simulink model "ques5"  (R2022b)
settings: Solver=ode4  StartTime=0.0  StopTime=10.0  FixedStep=0.0001  MaxStep=0.0001  RelTol=1e-3
values from neighbouring files (symbols this model uses):
  A = [a-b, 0.5-c; 0, 1]    [A2_2_4.m]    (also in A2_2_4_fin.m; A2_3_4_fin.m; A2_4_2.m = [a-bl, 0.5-c; 0, 1]; KA2_4.m = [a-bl, 0.5-c; 0, 1])
  B = [0; 1]    [A2_2_4.m]    (also in A2_2_4_fin.m; A2_3_4_fin.m; A2_4_2.m; KA2_4.m)
undefined symbols (not defined in the file or in its folder): C, D
settings Model: Creator=long  LastModifiedBy=munjunhwi
settings SolverCC: AlgebraicLoopSolver=TrustRegion
settings DebuggingCC: UnconnectedInputMsg=warning  UnconnectedOutputMsg=warning  UnconnectedLineMsg=warning  SFMachineParentedDataDiag=warning
settings ModelReferenceCC: EnableRefExpFcnMdlSchedulingChecks=on
settings RTWCC: DLArmComputeVersion=19.05

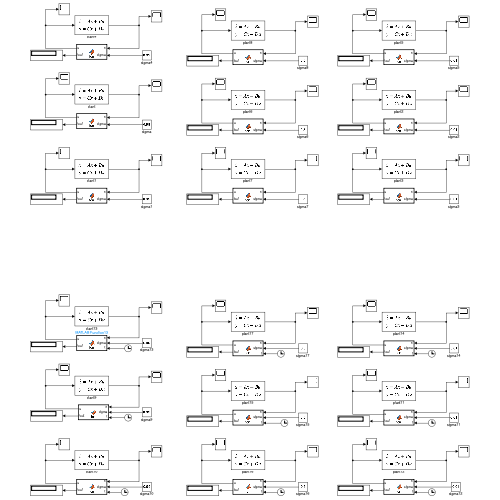
[thumbnail: Simulink's stored preview of the top-level diagram]
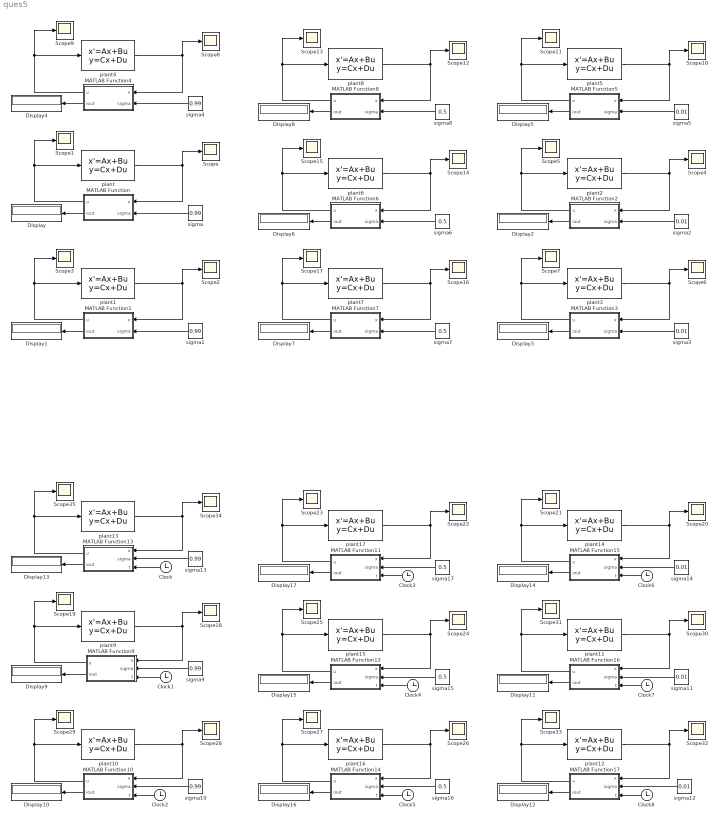
== system ques5 ==
  Clock{,1..8} (9 alike) : Clock
  Display{,1..17} (18 alike) : Display
  MATLAB Function : MATLAB Function  TreatAsAtomicUnit=on
  MATLAB Function1 : MATLAB Function  TreatAsAtomicUnit=on
  MATLAB Function10 : MATLAB Function  TreatAsAtomicUnit=on
  MATLAB Function11 : MATLAB Function  TreatAsAtomicUnit=on
  MATLAB Function12 : MATLAB Function  TreatAsAtomicUnit=on
  MATLAB Function13 : MATLAB Function  TreatAsAtomicUnit=on
  MATLAB Function14 : MATLAB Function  TreatAsAtomicUnit=on
  MATLAB Function15 : MATLAB Function  TreatAsAtomicUnit=on
  MATLAB Function16 : MATLAB Function  TreatAsAtomicUnit=on
  MATLAB Function17 : MATLAB Function  TreatAsAtomicUnit=on
  MATLAB Function2 : MATLAB Function  TreatAsAtomicUnit=on
  MATLAB Function3 : MATLAB Function  TreatAsAtomicUnit=on
  MATLAB Function4 : MATLAB Function  TreatAsAtomicUnit=on
  MATLAB Function5 : MATLAB Function  TreatAsAtomicUnit=on
  MATLAB Function6 : MATLAB Function  TreatAsAtomicUnit=on
  MATLAB Function7 : MATLAB Function  TreatAsAtomicUnit=on
  MATLAB Function8 : MATLAB Function  TreatAsAtomicUnit=on
  MATLAB Function9 : MATLAB Function  TreatAsAtomicUnit=on
  Scope{,1..35} (36 alike) : Scope
  plant{,2,6,9,11,15} (6 alike) : StateSpace  A=A  B=B  C=C  D=D  InitialCondition=[10;10]
  plant{1,3,7,10,12,16} (6 alike) : StateSpace  A=A  B=B  C=C  D=D  InitialCondition=[1;0]
  plant{4..5,8,13..14,17} (6 alike) : StateSpace  A=A  B=B  C=C  D=D  InitialCondition=[100;150]
  sigma{,1,4,9..10,13} (6 alike) : Constant  Value=0.99
  sigma{2..3,5,11..12,14} (6 alike) : Constant  Value=0.01
  sigma{6..8,15..17} (6 alike) : Constant  Value=0.5
  wires:
  sigma/1 -> MATLAB Function/2(sigma)
  plant/1 -> MATLAB Function/1(x), Scope/1
  MATLAB Function/1(u) -> Scope1/1, plant/1
  MATLAB Function/2(iout) -> Display/1
  MATLAB Function1/2(iout) -> Display1/1
  MATLAB Function1/1(u) -> Scope3/1, plant1/1
  sigma1/1 -> MATLAB Function1/2(sigma)
  plant1/1 -> MATLAB Function1/1(x), Scope2/1
  MATLAB Function2/2(iout) -> Display2/1
  MATLAB Function2/1(u) -> Scope5/1, plant2/1
  sigma2/1 -> MATLAB Function2/2(sigma)
  plant2/1 -> MATLAB Function2/1(x), Scope4/1
  MATLAB Function3/2(iout) -> Display3/1
  MATLAB Function3/1(u) -> Scope7/1, plant3/1
  sigma3/1 -> MATLAB Function3/2(sigma)
  plant3/1 -> MATLAB Function3/1(x), Scope6/1
  sigma5/1 -> MATLAB Function5/2(sigma)
  MATLAB Function5/1(u) -> Scope11/1, plant5/1
  MATLAB Function4/2(iout) -> Display4/1
  MATLAB Function4/1(u) -> Scope9/1, plant4/1
  sigma4/1 -> MATLAB Function4/2(sigma)
  plant5/1 -> MATLAB Function5/1(x), Scope10/1
  MATLAB Function5/2(iout) -> Display5/1
  plant4/1 -> MATLAB Function4/1(x), Scope8/1
  sigma6/1 -> MATLAB Function6/2(sigma)
  MATLAB Function6/1(u) -> Scope15/1, plant6/1
  plant6/1 -> MATLAB Function6/1(x), Scope14/1
  MATLAB Function8/1(u) -> Scope13/1, plant8/1
  MATLAB Function8/2(iout) -> Display8/1
  plant8/1 -> MATLAB Function8/1(x), Scope12/1
  MATLAB Function6/2(iout) -> Display6/1
  sigma8/1 -> MATLAB Function8/2(sigma)
  sigma7/1 -> MATLAB Function7/2(sigma)
  MATLAB Function7/1(u) -> Scope17/1, plant7/1
  plant7/1 -> MATLAB Function7/1(x), Scope16/1
  MATLAB Function7/2(iout) -> Display7/1
  sigma11/1 -> MATLAB Function16/2(sigma)
  MATLAB Function16/1(u) -> Scope31/1, plant11/1
  plant11/1 -> MATLAB Function16/1(x), Scope30/1
  MATLAB Function10/2(iout) -> Display10/1
  sigma10/1 -> MATLAB Function10/2(sigma)
  plant10/1 -> MATLAB Function10/1(x), Scope28/1
  MATLAB Function15/1(u) -> Scope21/1, plant14/1
  MATLAB Function13/2(iout) -> Display13/1
  MATLAB Function13/1(u) -> Scope35/1, plant13/1
  plant14/1 -> MATLAB Function15/1(x), Scope20/1
  MATLAB Function16/2(iout) -> Display11/1
  MATLAB Function17/1(u) -> Scope33/1, plant12/1
  sigma12/1 -> MATLAB Function17/2(sigma)
  MATLAB Function17/2(iout) -> Display12/1
  plant12/1 -> MATLAB Function17/1(x), Scope32/1
  MATLAB Function14/2(iout) -> Display16/1
  plant16/1 -> MATLAB Function14/1(x), Scope26/1
  MATLAB Function12/2(iout) -> Display15/1
  sigma16/1 -> MATLAB Function14/2(sigma)
  plant17/1 -> MATLAB Function11/1(x), Scope22/1
  sigma14/1 -> MATLAB Function15/2(sigma)
  MATLAB Function14/1(u) -> Scope27/1, plant16/1
  MATLAB Function10/1(u) -> Scope29/1, plant10/1
  plant15/1 -> MATLAB Function12/1(x), Scope24/1
  MATLAB Function12/1(u) -> Scope25/1, plant15/1
  sigma13/1 -> MATLAB Function13/2(sigma)
  MATLAB Function11/2(iout) -> Display17/1
  MATLAB Function11/1(u) -> Scope23/1, plant17/1
  sigma17/1 -> MATLAB Function11/2(sigma)
  MATLAB Function9/1(u) -> Scope19/1, plant9/1
  MATLAB Function9/2(iout) -> Display9/1
  MATLAB Function15/2(iout) -> Display14/1
  sigma9/1 -> MATLAB Function9/2(sigma)
  plant9/1 -> MATLAB Function9/1(x), Scope18/1
  sigma15/1 -> MATLAB Function12/2(sigma)
  plant13/1 -> MATLAB Function13/1(x), Scope34/1
  Clock/1 -> MATLAB Function13/3(t)
  Clock1/1 -> MATLAB Function9/3(t)
  Clock2/1 -> MATLAB Function10/3(t)
  Clock3/1 -> MATLAB Function11/3(t)
  Clock4/1 -> MATLAB Function12/3(t)
  Clock5/1 -> MATLAB Function14/3(t)
  Clock6/1 -> MATLAB Function15/3(t)
  Clock7/1 -> MATLAB Function16/3(t)
  Clock8/1 -> MATLAB Function17/3(t)

== matlab function ques5/MATLAB Function10 ==
  settings: updateMethod=DISCRETE
  data: x input; u output; sigma input; iout output; t input
function [u,iout]= fcn(x,sigma,t)
    persistent uk xk i;
    k1=zeros(1,2);
    A=zeros(2);
    B=zeros(2,1);
    P=zeros(2);
    Q=zeros(2);
    coder.extrinsic('evalin');
    A = evalin('base', 'A'); 
    B = evalin('base', 'B'); 
    P = evalin('base', 'P'); 
    Q = evalin('base', 'Q'); 
    k1 = evalin('base', 'k1'); 
    
    
    if isempty(uk)||isempty(xk)
        i=0;
        xk = x;
        uk=-k1*x;
    end

    
    if rem(t,0.0035)==0
        if [x' xk']*[A'*P+P*A+sigma*Q -P*B*k1;-(B*k1)'*P zeros(2)]*[x;xk]>=0
            i = i+1;
            uk = -k1*x;
            xk = x;
        end
    end

    u=uk;
    iout=i;
end

== matlab function ques5/MATLAB Function11 ==
  settings: updateMethod=DISCRETE
  data: x input; u output; sigma input; iout output; t input
function [u,iout]= fcn(x,sigma,t)
    persistent uk xk i;
    k1=zeros(1,2);
    A=zeros(2);
    B=zeros(2,1);
    P=zeros(2);
    Q=zeros(2);
    coder.extrinsic('evalin');
    A = evalin('base', 'A'); 
    B = evalin('base', 'B'); 
    P = evalin('base', 'P'); 
    Q = evalin('base', 'Q'); 
    k1 = evalin('base', 'k1'); 
    
    
    if isempty(uk)||isempty(xk)
        i=0;
        xk = x;
        uk=-k1*x;
    end

    
    if rem(t,0.0035)==0
        if [x' xk']*[A'*P+P*A+sigma*Q -P*B*k1;-(B*k1)'*P zeros(2)]*[x;xk]>=0
            i = i+1;
            uk = -k1*x;
            xk = x;
        end
    end

    u=uk;
    iout=i;
end

== matlab function ques5/MATLAB Function13 ==
  settings: updateMethod=DISCRETE
  data: x input; u output; sigma input; iout output; t input
function [u,iout]= fcn(x,sigma,t)
    persistent uk xk i;
    k1=zeros(1,2);
    A=zeros(2);
    B=zeros(2,1);
    P=zeros(2);
    Q=zeros(2);
    coder.extrinsic('evalin');
    A = evalin('base', 'A'); 
    B = evalin('base', 'B'); 
    P = evalin('base', 'P'); 
    Q = evalin('base', 'Q'); 
    k1 = evalin('base', 'k1'); 
    
    
    if isempty(uk)||isempty(xk)
        i=0;
        xk = x;
        uk=-k1*x;
    end

    
    if rem(t,0.0035)==0 %sampling time 0.0035
        if [x' xk']*[A'*P+P*A+sigma*Q -P*B*k1;-(B*k1)'*P zeros(2)]*[x;xk]>=0
            i = i+1;
            uk = -k1*x;
            xk = x;
        end
    end

    u=uk;
    iout=i;
end

== matlab function ques5/MATLAB Function12 ==
  settings: updateMethod=DISCRETE
  data: x input; u output; sigma input; iout output; t input
function [u,iout]= fcn(x,sigma,t)
    persistent uk xk i;
    k1=zeros(1,2);
    A=zeros(2);
    B=zeros(2,1);
    P=zeros(2);
    Q=zeros(2);
    coder.extrinsic('evalin');
    A = evalin('base', 'A'); 
    B = evalin('base', 'B'); 
    P = evalin('base', 'P'); 
    Q = evalin('base', 'Q'); 
    k1 = evalin('base', 'k1'); 
    
    
    if isempty(uk)||isempty(xk)
        i=0;
        xk = x;
        uk=-k1*x;
    end

    
    if rem(t,0.0035)==0
        if [x' xk']*[A'*P+P*A+sigma*Q -P*B*k1;-(B*k1)'*P zeros(2)]*[x;xk]>=0
            i = i+1;
            uk = -k1*x;
            xk = x;
        end
    end

    u=uk;
    iout=i;
end

== matlab function ques5/MATLAB Function14 ==
  settings: updateMethod=DISCRETE
  data: x input; u output; sigma input; iout output; t input
function [u,iout]= fcn(x,sigma,t)
    persistent uk xk i;
    k1=zeros(1,2);
    A=zeros(2);
    B=zeros(2,1);
    P=zeros(2);
    Q=zeros(2);
    coder.extrinsic('evalin');
    A = evalin('base', 'A'); 
    B = evalin('base', 'B'); 
    P = evalin('base', 'P'); 
    Q = evalin('base', 'Q'); 
    k1 = evalin('base', 'k1'); 
    
    
    if isempty(uk)||isempty(xk)
        i=0;
        xk = x;
        uk=-k1*x;
    end

    
    if rem(t,0.0035)==0
        if [x' xk']*[A'*P+P*A+sigma*Q -P*B*k1;-(B*k1)'*P zeros(2)]*[x;xk]>=0
            i = i+1;
            uk = -k1*x;
            xk = x;
        end
    end

    u=uk;
    iout=i;
end

== matlab function ques5/MATLAB Function15 ==
  settings: updateMethod=DISCRETE
  data: x input; u output; sigma input; iout output; t input
function [u,iout]= fcn(x,sigma,t)
    persistent uk xk i;
    k1=zeros(1,2);
    A=zeros(2);
    B=zeros(2,1);
    P=zeros(2);
    Q=zeros(2);
    coder.extrinsic('evalin');
    A = evalin('base', 'A'); 
    B = evalin('base', 'B'); 
    P = evalin('base', 'P'); 
    Q = evalin('base', 'Q'); 
    k1 = evalin('base', 'k1'); 
    
    
    if isempty(uk)||isempty(xk)
        i=0;
        xk = x;
        uk=-k1*x;
    end

    
    if rem(t,0.0035)==0
        if [x' xk']*[A'*P+P*A+sigma*Q -P*B*k1;-(B*k1)'*P zeros(2)]*[x;xk]>=0
            i = i+1;
            uk = -k1*x;
            xk = x;
        end
    end

    u=uk;
    iout=i;
end

== matlab function ques5/MATLAB Function1 ==
  settings: updateMethod=DISCRETE
  data: x input; u output; sigma input; iout output
function [u,iout]= fcn(x,sigma)
    persistent uk xk i;
    k1=zeros(1,2);
    A=zeros(2);
    B=zeros(2,1);
    P=zeros(2);
    Q=zeros(2);
    coder.extrinsic('evalin');
    A = evalin('base', 'A'); 
    B = evalin('base', 'B'); 
    P = evalin('base', 'P'); 
    Q = evalin('base', 'Q'); 
    k1 = evalin('base', 'k1'); 
    
    
    if isempty(uk)||isempty(xk)
        i=0;
        xk = x;
        uk=-k1*x;
    end

    if [x' xk']*[A'*P+P*A+sigma*Q -P*B*k1;-(B*k1)'*P zeros(2)]*[x;xk]>=0
        i = i+1;
        uk = -k1*x;
        xk = x;
    end

    u=uk;
    iout=i;
end

== matlab function ques5/MATLAB Function16 ==
  settings: updateMethod=DISCRETE
  data: x input; u output; sigma input; iout output; t input
function [u,iout]= fcn(x,sigma,t)
    persistent uk xk i;
    k1=zeros(1,2);
    A=zeros(2);
    B=zeros(2,1);
    P=zeros(2);
    Q=zeros(2);
    coder.extrinsic('evalin');
    A = evalin('base', 'A'); 
    B = evalin('base', 'B'); 
    P = evalin('base', 'P'); 
    Q = evalin('base', 'Q'); 
    k1 = evalin('base', 'k1'); 
    
    
    if isempty(uk)||isempty(xk)
        i=0;
        xk = x;
        uk=-k1*x;
    end

    
    if rem(t,0.0035)==0
        if [x' xk']*[A'*P+P*A+sigma*Q -P*B*k1;-(B*k1)'*P zeros(2)]*[x;xk]>=0
            i = i+1;
            uk = -k1*x;
            xk = x;
        end
    end

    u=uk;
    iout=i;
end

== matlab function ques5/MATLAB Function17 ==
  settings: updateMethod=DISCRETE
  data: x input; u output; sigma input; iout output; t input
function [u,iout]= fcn(x,sigma,t)
    persistent uk xk i;
    k1=zeros(1,2);
    A=zeros(2);
    B=zeros(2,1);
    P=zeros(2);
    Q=zeros(2);
    coder.extrinsic('evalin');
    A = evalin('base', 'A'); 
    B = evalin('base', 'B'); 
    P = evalin('base', 'P'); 
    Q = evalin('base', 'Q'); 
    k1 = evalin('base', 'k1'); 
    
    
    if isempty(uk)||isempty(xk)
        i=0;
        xk = x;
        uk=-k1*x;
    end

    
    if rem(t,0.0035)==0
        if [x' xk']*[A'*P+P*A+sigma*Q -P*B*k1;-(B*k1)'*P zeros(2)]*[x;xk]>=0
            i = i+1;
            uk = -k1*x;
            xk = x;
        end
    end

    u=uk;
    iout=i;
end

== matlab function ques5/MATLAB Function ==
  settings: updateMethod=DISCRETE
  data: x input; u output; sigma input; iout output
function [u,iout]= fcn(x,sigma)
    persistent uk xk i;
    k1=zeros(1,2);
    A=zeros(2);
    B=zeros(2,1);
    P=zeros(2);
    Q=zeros(2);
    coder.extrinsic('evalin');
    A = evalin('base', 'A'); 
    B = evalin('base', 'B'); 
    P = evalin('base', 'P'); 
    Q = evalin('base', 'Q'); 
    k1 = evalin('base', 'k1'); 
    
    
    if isempty(uk)||isempty(xk)
        i=0;
        xk = x;
        uk=-k1*x;
    end

    if [x' xk']*[A'*P+P*A+sigma*Q -P*B*k1;-(B*k1)'*P zeros(2)]*[x;xk]>=0
        i = i+1;
        uk = -k1*x;
        xk = x;
    end

    u=uk;
    iout=i;
end

== matlab function ques5/MATLAB Function2 ==
  settings: updateMethod=DISCRETE
  data: x input; u output; sigma input; iout output
function [u,iout]= fcn(x,sigma)
    persistent uk xk i;
    k1=zeros(1,2);
    A=zeros(2);
    B=zeros(2,1);
    P=zeros(2);
    Q=zeros(2);
    coder.extrinsic('evalin');
    A = evalin('base', 'A'); 
    B = evalin('base', 'B'); 
    P = evalin('base', 'P'); 
    Q = evalin('base', 'Q'); 
    k1 = evalin('base', 'k1'); 
    
    
    if isempty(uk)||isempty(xk)
        i=0;
        xk = x;
        uk=-k1*x;
    end

    if [x' xk']*[A'*P+P*A+sigma*Q -P*B*k1;-(B*k1)'*P zeros(2)]*[x;xk]>=0
        i = i+1;
        uk = -k1*x;
        xk = x;
    end

    u=uk;
    iout=i;
end

== matlab function ques5/MATLAB Function3 ==
  settings: updateMethod=DISCRETE
  data: x input; u output; sigma input; iout output
function [u,iout]= fcn(x,sigma)
    persistent uk xk i;
    k1=zeros(1,2);
    A=zeros(2);
    B=zeros(2,1);
    P=zeros(2);
    Q=zeros(2);
    coder.extrinsic('evalin');
    A = evalin('base', 'A'); 
    B = evalin('base', 'B'); 
    P = evalin('base', 'P'); 
    Q = evalin('base', 'Q'); 
    k1 = evalin('base', 'k1'); 
    
    
    if isempty(uk)||isempty(xk)
        i=0;
        xk = x;
        uk=-k1*x;
    end

    if [x' xk']*[A'*P+P*A+sigma*Q -P*B*k1;-(B*k1)'*P zeros(2)]*[x;xk]>=0
        i = i+1;
        uk = -k1*x;
        xk = x;
    end

    u=uk;
    iout=i;
end

== matlab function ques5/MATLAB Function4 ==
  settings: updateMethod=DISCRETE
  data: x input; u output; sigma input; iout output
function [u,iout]= fcn(x,sigma)
    persistent uk xk i;
    k1=zeros(1,2);
    A=zeros(2);
    B=zeros(2,1);
    P=zeros(2);
    Q=zeros(2);
    coder.extrinsic('evalin');
    A = evalin('base', 'A'); 
    B = evalin('base', 'B'); 
    P = evalin('base', 'P'); 
    Q = evalin('base', 'Q'); 
    k1 = evalin('base', 'k1'); 
    
    
    if isempty(uk)||isempty(xk)
        i=0;
        xk = x;
        uk=-k1*x;
    end

    if [x' xk']*[A'*P+P*A+sigma*Q -P*B*k1;-(B*k1)'*P zeros(2)]*[x;xk]>=0
        i = i+1;
        uk = -k1*x;
        xk = x;
    end

    u=uk;
    iout=i;
end

== matlab function ques5/MATLAB Function5 ==
  settings: updateMethod=DISCRETE
  data: x input; u output; sigma input; iout output
function [u,iout]= fcn(x,sigma)
    persistent uk xk i;
    k1=zeros(1,2);
    A=zeros(2);
    B=zeros(2,1);
    P=zeros(2);
    Q=zeros(2);
    coder.extrinsic('evalin');
    A = evalin('base', 'A'); 
    B = evalin('base', 'B'); 
    P = evalin('base', 'P'); 
    Q = evalin('base', 'Q'); 
    k1 = evalin('base', 'k1'); 
    
    
    if isempty(uk)||isempty(xk)
        i=0;
        xk = x;
        uk=-k1*x;
    end

    if [x' xk']*[A'*P+P*A+sigma*Q -P*B*k1;-(B*k1)'*P zeros(2)]*[x;xk]>=0
        i = i+1;
        uk = -k1*x;
        xk = x;
    end

    u=uk;
    iout=i;
end

== matlab function ques5/MATLAB Function6 ==
  settings: updateMethod=DISCRETE
  data: x input; u output; sigma input; iout output
function [u,iout]= fcn(x,sigma)
    persistent uk xk i;
    k1=zeros(1,2);
    A=zeros(2);
    B=zeros(2,1);
    P=zeros(2);
    Q=zeros(2);
    coder.extrinsic('evalin');
    A = evalin('base', 'A'); 
    B = evalin('base', 'B'); 
    P = evalin('base', 'P'); 
    Q = evalin('base', 'Q'); 
    k1 = evalin('base', 'k1'); 
    
    
    if isempty(uk)||isempty(xk)
        i=0;
        xk = x;
        uk=-k1*x;
    end

    if [x' xk']*[A'*P+P*A+sigma*Q -P*B*k1;-(B*k1)'*P zeros(2)]*[x;xk]>=0
        i = i+1;
        uk = -k1*x;
        xk = x;
    end

    u=uk;
    iout=i;
end

== matlab function ques5/MATLAB Function7 ==
  settings: updateMethod=DISCRETE
  data: x input; u output; sigma input; iout output
function [u,iout]= fcn(x,sigma)
    persistent uk xk i;
    k1=zeros(1,2);
    A=zeros(2);
    B=zeros(2,1);
    P=zeros(2);
    Q=zeros(2);
    coder.extrinsic('evalin');
    A = evalin('base', 'A'); 
    B = evalin('base', 'B'); 
    P = evalin('base', 'P'); 
    Q = evalin('base', 'Q'); 
    k1 = evalin('base', 'k1'); 
    
    
    if isempty(uk)||isempty(xk)
        i=0;
        xk = x;
        uk=-k1*x;
    end

    if [x' xk']*[A'*P+P*A+sigma*Q -P*B*k1;-(B*k1)'*P zeros(2)]*[x;xk]>=0
        i = i+1;
        uk = -k1*x;
        xk = x;
    end

    u=uk;
    iout=i;
end

== matlab function ques5/MATLAB Function8 ==
  settings: updateMethod=DISCRETE
  data: x input; u output; sigma input; iout output
function [u,iout]= fcn(x,sigma)
    persistent uk xk i;
    k1=zeros(1,2);
    A=zeros(2);
    B=zeros(2,1);
    P=zeros(2);
    Q=zeros(2);
    coder.extrinsic('evalin');
    A = evalin('base', 'A'); 
    B = evalin('base', 'B'); 
    P = evalin('base', 'P'); 
    Q = evalin('base', 'Q'); 
    k1 = evalin('base', 'k1'); 
    
    
    if isempty(uk)||isempty(xk)
        i=0;
        xk = x;
        uk=-k1*x;
    end

    if [x' xk']*[A'*P+P*A+sigma*Q -P*B*k1;-(B*k1)'*P zeros(2)]*[x;xk]>=0
        i = i+1;
        uk = -k1*x;
        xk = x;
    end

    u=uk;
    iout=i;
end

== matlab function ques5/MATLAB Function9 ==
  settings: updateMethod=DISCRETE
  data: x input; u output; sigma input; iout output; t input
function [u,iout]= fcn(x,sigma,t)
    persistent uk xk i;
    k1=zeros(1,2);
    A=zeros(2);
    B=zeros(2,1);
    P=zeros(2);
    Q=zeros(2);
    coder.extrinsic('evalin');
    A = evalin('base', 'A'); 
    B = evalin('base', 'B'); 
    P = evalin('base', 'P'); 
    Q = evalin('base', 'Q'); 
    k1 = evalin('base', 'k1'); 
    
    
    if isempty(uk)||isempty(xk)
        i=0;
        xk = x;
        uk=-k1*x;
    end

    
    if rem(t,0.0035)==0
        if [x' xk']*[A'*P+P*A+sigma*Q -P*B*k1;-(B*k1)'*P zeros(2)]*[x;xk]>=0
            i = i+1;
            uk = -k1*x;
            xk = x;
        end
    end

    u=uk;
    iout=i;
end
